simulink model "Cartesian_Regulation"  (R2022b)
settings: Solver=FixedStepAuto  StartTime=0.0  StopTime=10.0  MaxStep=0.1  RelTol=1e-3
undefined symbols (not defined in the file): K_v, K_w, theta_i, x_f, x_i, y_f, y_i
libraries: simulink_extras x1
settings Model: Creator=hp 2021  LastModifiedBy=Musta
settings ModelReferenceCC: EnableRefExpFcnMdlSchedulingChecks=on

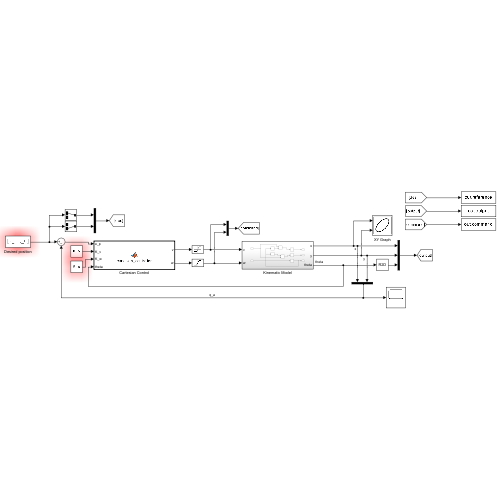
[thumbnail: Simulink's stored preview of the top-level diagram]
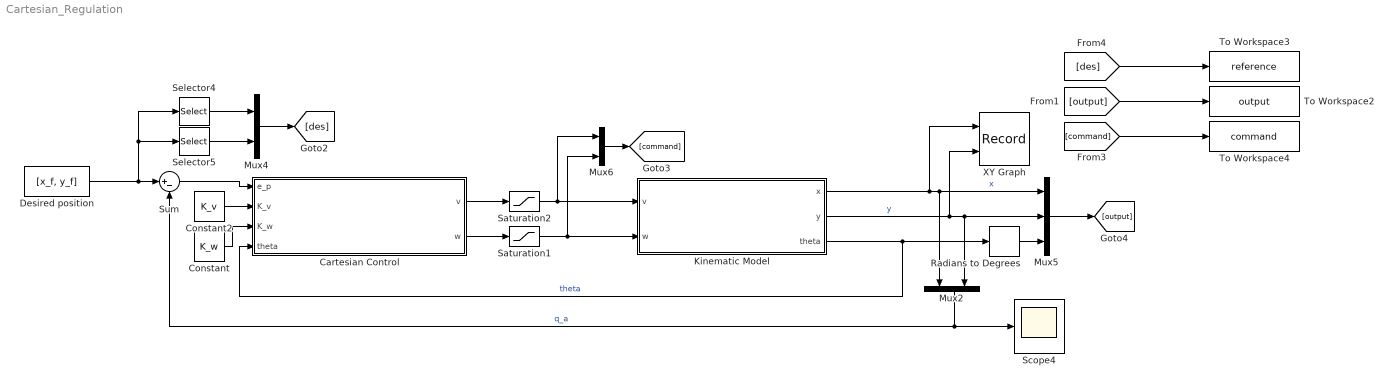
== system Cartesian_Regulation ==
  Cartesian Control : MATLAB Function  TreatAsAtomicUnit=on
  Constant : Constant  Value=K_w
  Constant2 : Constant  Value=K_v
  Desired position : Constant  Value=[x_f, y_f]
  Kinematic Model : Subsystem
  Mux2 : Mux  Inputs=2
  Mux4 : Mux  Inputs=2
  Mux5 : Mux  Inputs=3
  Mux6 : Mux  Inputs=2
  Radians to Degrees : simulink_extras/Transformations/Radians to Degrees
  Saturation1 : Saturate  UpperLimit=2  LowerLimit=-2
  Saturation2 : Saturate  UpperLimit=2  LowerLimit=-2
  Scope4 : Scope
  Selector4 : Selector  InputPortWidth=2  IndexOptions=Index vector (dialog)  Indices=1  OutputSizes=1
  Selector5 : Selector  InputPortWidth=2  IndexOptions=Index vector (dialog)  Indices=2  OutputSizes=1
  Sum : Sum  Inputs=|+-
  To Workspace2 : ToWorkspace  VariableName=output  SaveFormat=Structure With Time  SampleTime=-1
  To Workspace3 : ToWorkspace  VariableName=reference  SaveFormat=Structure With Time  SampleTime=-1
  To Workspace4 : ToWorkspace  VariableName=command  SaveFormat=Structure With Time  SampleTime=-1
  XY Graph : Record  FileSettingsInternal="{\"entries\":[{\"content\":{\"excelSettings\":{\"content\":{},\"type\":\"Streamout.ExcelSettings\"}},\"type\":\"Streamout.FileSettingStorage\",\"uuid\":\"966b7fe5-a256-4086-963b-c256e5ee5b6b\"}],\"packageUris\":[\"http://schema.mathworks.com/mf0/streamout_blocks/R2020a\"],\"version\":\"1.0\"}"  Layout=[1 1]  SignalsInternal="{\"entries\":[{\"content\":{\"signals\":[{\"content\":{\"blockPath\":[\"Cartesian_Regulation/XY Graph2\"],\"channel\":[],\"dimensions\":[1],\"domain\":\"Cartesian_Regulation/XY Graph2\",\"lineColor\":\"#a2142f\",\"plots\":[1],\"port\":1,\"sid\":[],\"signalID\":8,\"signalName\":\"x\"},\"type\":\"RecordBlkView.Signal\",\"uuid\":\"054d6c21-b5c4-4ca3-a6b3-d04dc938c854\"},{\"content\":{\"blockPath\":[\"Cartesian_Regulation/XY Graph2\"],\"channel\":[],\"dimensions\":[1],\"domain\":\"Cartesian_Regulation/XY Graph2\",\"lineColor\":\"#139fff\",\"plots\":[1],\"port\":2,\"sid\":[],\"signalID\":11,\"signalName\":\"y\"},\"type\":\"RecordBlkView.Signal\",\"uuid\":\"244c9a56-8795-4af3-9f78-fc3e758ed6f6\"}]},\"type\":\"RecordBlkView.InputSignals\",\"uuid\":\"6dca512b-0974-4d29-b675-5ca2ca014814\"}],\"packageUris\":[\"http://schema.mathworks.com/mf0/streamout_blocks/R2020a\"],\"version\":\"1.0\"}"  VisualizationBindings="{\"xyplotplugin\":{\"info\":[{\"series\":[{\"bindingParametersList\":[{\"parameter\":\"X-Axis\",\"signalID\":8,\"signalName\":\"x\"},{\"parameter\":\"Y-Axis\",\"signalID\":11,\"signalName\":\"y\"}],\"seriesID\":61401}],\"subplotID\":1}]}}"  CompatibilityTag=XY
  wires:
  Cartesian Control/1(v) -> Saturation2/1
  Desired position/1 -> Sum/1, Selector4/1, Selector5/1
  Mux5/1 -> [output]
  Selector5/1 -> Mux4/2
  Mux6/1 -> [command]
  Saturation2/1 -> Kinematic Model/1(v), Mux6/1
  Kinematic Model/1(x) -> Mux2/1, Mux5/1, XY Graph/1  "x"
  Kinematic Model/3(theta) -> Cartesian Control/4(theta), Radians to Degrees/1  "theta"
  Cartesian Control/2(w) -> Saturation1/1
  Selector4/1 -> Mux4/1
  [command] -> To Workspace4/1
  Saturation1/1 -> Mux6/2, Kinematic Model/2(w)
  Radians to Degrees/1 -> Mux5/3
  Mux4/1 -> [des]
  [output] -> To Workspace2/1
  [des] -> To Workspace3/1
  Mux2/1 -> Sum/2, Scope4/1  "q_a"
  Kinematic Model/2(y) -> XY Graph/2, Mux5/2, Mux2/2  "y"
  Constant2/1 -> Cartesian Control/2(K_v)
  Sum/1 -> Cartesian Control/1(e_p)
  Constant/1 -> Cartesian Control/3(K_w)

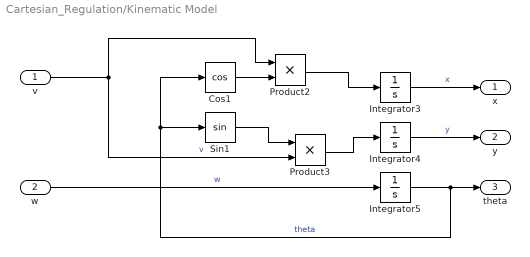
== system Cartesian_Regulation/Kinematic Model ==
  v : Inport
  w : Inport  Port=2
  Cos1 : Trigonometry  Operator=cos
  Integrator3 : Integrator  InitialCondition=x_i
  Integrator4 : Integrator  InitialCondition=y_i
  Integrator5 : Integrator  InitialCondition=theta_i
  Product2 : Product
  Product3 : Product
  Sin1 : Trigonometry
  x : Outport
  y : Outport  Port=2
  theta : Outport  Port=3
  wires:
  Integrator3/1 -> x/1  "x"
  Integrator4/1 -> y/1  "y"
  Cos1/1 -> Product2/2
  Product3/1 -> Integrator4/1
  Integrator5/1 -> Cos1/1, Sin1/1, theta/1  "theta"
  Product2/1 -> Integrator3/1
  v/1 -> Product2/1, Product3/2  "v"
  Sin1/1 -> Product3/1
  w/1 -> Integrator5/1  "w"

== matlab function Cartesian_Regulation/Cartesian Control ==
  data: v output; w output; e_p input; K_v input; K_w input; theta input
function [v,w] = cartesian_controller(e_p, K_v, K_w, theta)

    v = K_v * (e_p(1)*cos(theta) + e_p(2)*sin(theta));
    w = K_w * (atan2(e_p(2),e_p(1))- theta);

end
